simulink model "poscontrol"  (R2015b)
settings: Solver=ode4  StartTime=0.0  StopTime=10  FixedStep=0.0002  RelTol=1e-3
values from neighbouring files (symbols this model uses):
  alpha = 1/K(1)    [lsrl.m]    (also in parameters.m = 66.9379)
  Kd = (2*zeta*omega+p-tau)/alpha    [parameters.m]
  Ki = (omega^2*p)/alpha    [parameters.m]
  Kp = (omega^2+2*zeta*omega*p)/alpha    [parameters.m]
  tau = alpha*K(2)    [lsrl.m]    (also in parameters.m = 39.3285)
settings Model: ExtModeTrigDuration=10000  Creator=flynng  LastModifiedBy=flynng
settings SolverCC: PositivePriorityOrder=on
settings RTWCC: SystemTargetFile=quarc_win64.tlc  TemplateMakefile=quarc_default_tmf  Description=QUARC Win64 Target
settings STFCustomTargetCC: TargetPreCompLibLocation=C:\ProgramData\QUARC\lib\2015b\win64\release  GeneratePreprocessorConditionals=Use local settings  CPPClassGenCompliant=off
settings GRTTargetCC: TargetPreCompLibLocation=C:\ProgramData\QUARC\lib\2015b\win64\release  ParMdlRefBuildCompliant=off  CompOptLevelCompliant=off  CombineOutputUpdateFcns=off  MatFileLogging=off  CPPClassGenCompliant=off  GRTInterface=on  UseToolchainInfoCompliant=off  ExtMode=on  ExtModeMexFile=quarc_comm

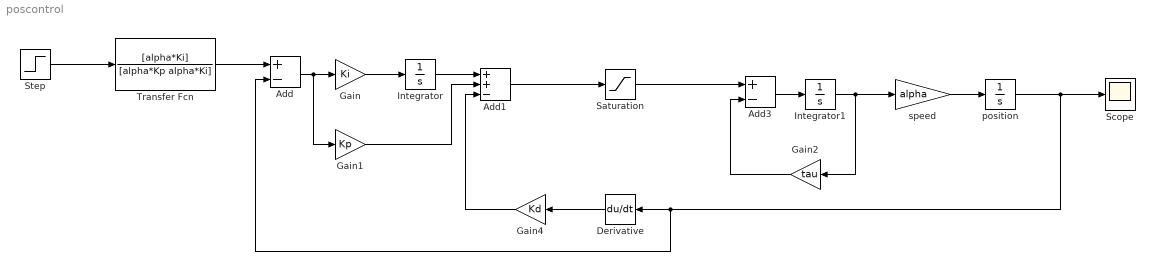
== system poscontrol ==
  Add : Sum  Inputs=+-
  Add1 : Sum  Inputs=++-
  Add3 : Sum  Inputs=+-
  Derivative : Derivative
  Gain : Gain  Gain=Ki
  Gain1 : Gain  Gain=Kp
  Gain2 : Gain  Gain=tau
  Gain4 : Gain  Gain=Kd
  Integrator : Integrator
  Integrator1 : Integrator
  Saturation : Saturate  UpperLimit=10  LowerLimit=-10
  Scope : Scope
  Step : Step  Time=0  SampleTime=0
  Transfer Fcn : TransferFcn  Numerator=[alpha*Ki]  Denominator=[alpha*Kp alpha*Ki]
  position : Integrator
  speed : Gain  Gain=alpha
  wires:
  Integrator1/1 -> speed/1, Gain2/1
  Gain2/1 -> Add3/2
  Add3/1 -> Integrator1/1
  Add1/1 -> Saturation/1
  Saturation/1 -> Add3/1
  Derivative/1 -> Gain4/1
  Gain4/1 -> Add1/3
  Add/1 -> Gain1/1, Gain/1
  Gain/1 -> Integrator/1
  Gain1/1 -> Add1/2
  Integrator/1 -> Add1/1
  speed/1 -> position/1
  position/1 -> Add/2, Derivative/1, Scope/1
  Transfer Fcn/1 -> Add/1
  Step/1 -> Transfer Fcn/1
